simulink model "Motion_control"  (R2021a)
settings: Solver=ode4  StartTime=0.0  StopTime=2+dt  FixedStep=0.001  RelTol=1e-3
settings Model: Creator=Ashut  LastModifiedBy=Ashut

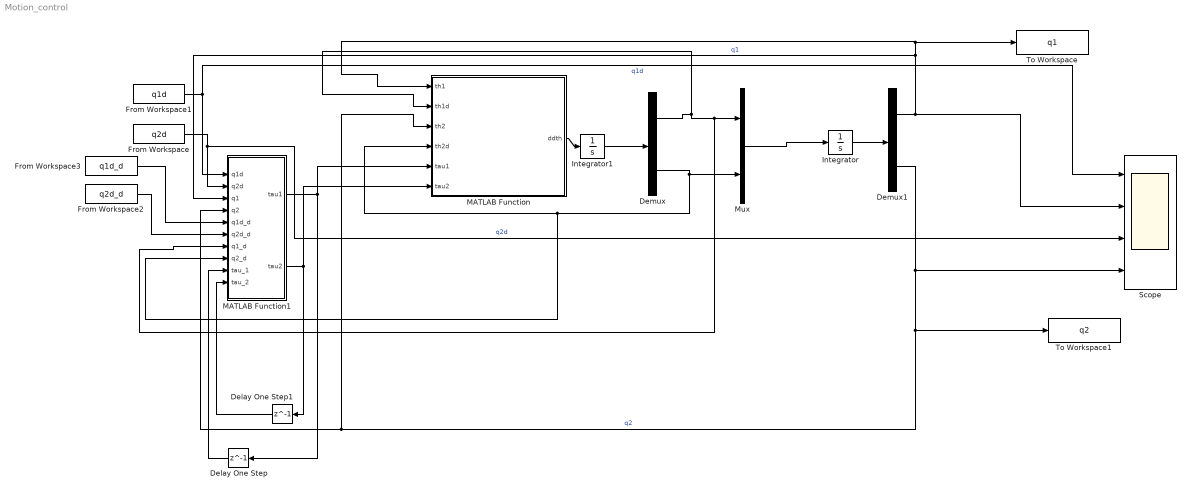
== system Motion_control ==
  Delay One Step : Delay  DelayLength=1
  Delay One Step1 : Delay  DelayLength=1
  Demux : Demux  Outputs=2
  Demux1 : Demux  Outputs=2
  From Workspace : FromWorkspace  VariableName=q2d
  From Workspace1 : FromWorkspace  VariableName=q1d
  From Workspace2 : FromWorkspace  VariableName=q2d_d
  From Workspace3 : FromWorkspace  VariableName=q1d_d
  Integrator : Integrator  InitialCondition=[0;0]
  Integrator1 : Integrator  InitialCondition=[0;0]
  MATLAB Function : MATLAB Function  TreatAsAtomicUnit=on
  MATLAB Function1 : MATLAB Function  TreatAsAtomicUnit=on
  Mux : Mux  Inputs=2
  Scope : Scope  NumInputPorts=4
  To Workspace : ToWorkspace  VariableName=q1  SaveFormat=Timeseries  SampleTime=-1
  To Workspace1 : ToWorkspace  VariableName=q2  SaveFormat=Timeseries  SampleTime=-1
  wires:
  Demux/1 -> MATLAB Function/2(th1d), MATLAB Function1/7(q1_d), Mux/1
  Demux/2 -> MATLAB Function1/8(q2_d), MATLAB Function/4(th2d), Mux/2
  Mux/1 -> Integrator/1
  Integrator/1 -> Demux1/1
  MATLAB Function/1(ddth) -> Integrator1/1
  Integrator1/1 -> Demux/1
  Demux1/1 -> MATLAB Function1/3(q1), MATLAB Function/1(th1), To Workspace/1, Scope/2  "q1"
  Demux1/2 -> MATLAB Function/3(th2), MATLAB Function1/4(q2), To Workspace1/1, Scope/4  "q2"
  MATLAB Function1/2(tau2) -> MATLAB Function/6(tau2), Delay One Step1/1
  MATLAB Function1/1(tau1) -> MATLAB Function/5(tau1), Delay One Step/1
  From Workspace/1 -> Scope/3, MATLAB Function1/2(q2d)  "q2d"
  From Workspace1/1 -> Scope/1, MATLAB Function1/1(q1d)  "q1d"
  Delay One Step/1 -> MATLAB Function1/9(tau_1)
  Delay One Step1/1 -> MATLAB Function1/10(tau_2)
  From Workspace3/1 -> MATLAB Function1/5(q1d_d)
  From Workspace2/1 -> MATLAB Function1/6(q2d_d)

== matlab function Motion_control/MATLAB Function1 ==
  data: q1d input; q2d input; tau1 output; q1 input; q2 input; tau2 output; q1d_d input; q2d_d input; q1_d input; q2_d input; tau_1 input; tau_2 input
function [tau1,tau2] = fcn(q1d,q2d,q1,q2,q1d_d,q2d_d,q1_d,q2_d,tau_1,tau_2)
Kp1= 0.1;
Kd1 = 10;
% dt=1/1000;
% t=0:dt:2+dt;
% tau1 = 0*t;
% tau2 = 0*t;
tau1 = tau_1 + Kp1*(q1d - q1)+Kd1*(q1d_d - q1_d);
tau2 = tau_2 + Kp1*(q2d - q2)+Kd1*(q2d_d - q2_d);

== matlab function Motion_control/MATLAB Function ==
  data: th1 input; th1d input; th2 input; th2d input; ddth output; tau1 input; tau2 input
function ddth= ode_solver_script_q1_a(th1,th1d,th2,th2d,tau1,tau2)
x = [th1;th1d;th2;th2d];
%% Input parameters
m2=1; m1=1; l1=1; l2=1; g=9.81;



%% Equation of motion 

%M matrix
M11=((((m1/3) + m2)*l1^2) +((m2/3)*l2^2) + (m2*l1*l2*cos(x(3))));
M12=(m2*(((l2^2)/3) + (0.5*l1*l2*cos(x(3)))));
M21=M12;
M22=((1/3)*m2*l2*l2);

%H matrix
H1 =((-m2*l1*l2*sin(x(3))*x(2)*x(4)) - (0.5*m2*l1*l2*sin(x(3))*x(4)*x(4)));
H2 = (0.5 * m2* l1*l2*sin(x(3))*x(2)*x(2));

%G matrix
G1=( ((((0.5*m1) + m2)*l1*cos(x(1))) + (0.5*m2*l2*cos(x(1)+x(3))))*g);
G2=0.5*m2*l2*cos(x(1)+x(3))*g;



M=[M11 M12;M21 M22];

HG = [H1 + G1; H2 + G2];

T=[tau1; tau2];

%% Equation in terms of acceleration

ddth = (inv(M)) * (T  - HG )    ;% Joint  accelaration
